simulink model "CP_DTSFC_Lin_b_n9945008"  (R2018b)
settings: Solver=FixedStepDiscrete  StartTime=0.0  StopTime=3  FixedStep=T_s  RelTol=1e-3
values from neighbouring files (symbols this model uses):
  Ad = sysdzoh.A    [CP_DTSFC_Lin_b_MainFile_n9945008.m]
  Bd = sysdzoh.B    [CP_DTSFC_Lin_b_MainFile_n9945008.m]
  Cd = sysdzoh.C    [CP_DTSFC_Lin_b_MainFile_n9945008.m]
  Dd = sysdzoh.D    [CP_DTSFC_Lin_b_MainFile_n9945008.m]
  K_db = place(sysdzoh.A ,sysdzoh.B ,dLambda)    [CP_DTSFC_Lin_b_MainFile_n9945008.m]
  T_s = 0.03    [CP_DTSFC_Lin_a_MainFile_n9945008.m]    (also in CP_DTSFC_Lin_b_MainFile_n9945008.m)
  x0 = [0.2 20*pi/180 0 0]'    [CP_DTSFC_Lin_a_MainFile_n9945008.m]    (also in CP_DTSFC_Lin_b_MainFile_n9945008.m)
settings Model: Creator=csmithcripps  LastModifiedBy=CodyS

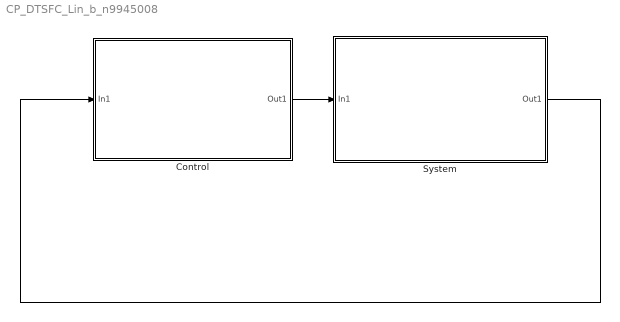
== system CP_DTSFC_Lin_b_n9945008 ==
  Control : Subsystem
  "System " : Subsystem
  wires:
  Control/1(Out1) -> "System "/1(In1)
  "System "/1(Out1) -> Control/1(In1)

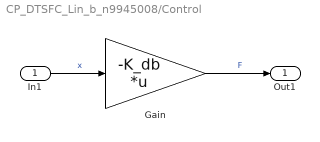
== system CP_DTSFC_Lin_b_n9945008/Control ==
  In1 : Inport
  Gain : Gain  Gain=-K_db  Multiplication=Matrix(K*u)
  Out1 : Outport
  wires:
  Gain/1 -> Out1/1  "F"
  In1/1 -> Gain/1  "x"

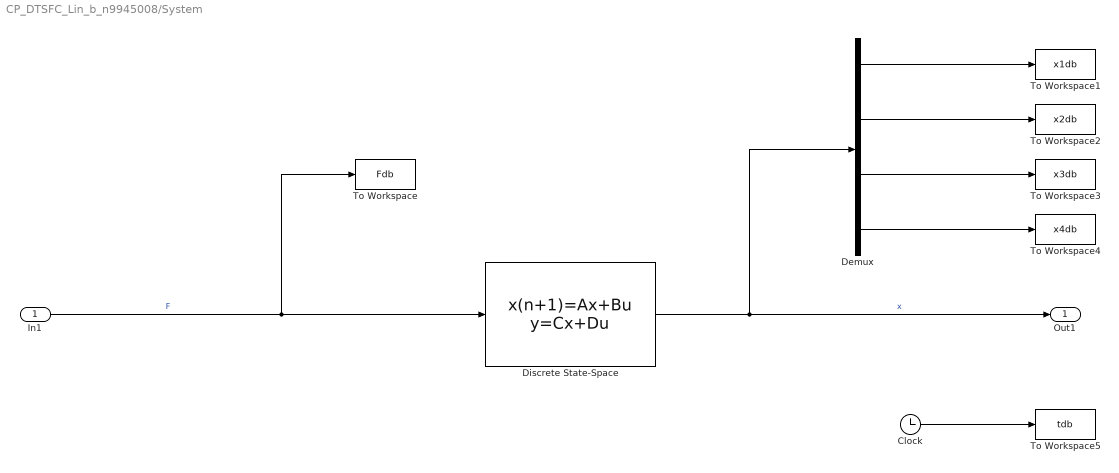
== system CP_DTSFC_Lin_b_n9945008/System  ==
  In1 : Inport
  Clock : Clock
  Demux : Demux
  Discrete State-Space : DiscreteStateSpace  A=Ad  B=Bd  C=Cd  D=Dd  InitialCondition=x0  SampleTime=T_s
  To Workspace : ToWorkspace  VariableName=Fdb  SampleTime=T_s
      settings: Save2DSignal=2-D array (concatenate along first dimension)
  To Workspace1 : ToWorkspace  VariableName=x1db  SampleTime=-1
      settings: Save2DSignal=2-D array (concatenate along first dimension)
  To Workspace2 : ToWorkspace  VariableName=x2db  SampleTime=-1
      settings: Save2DSignal=2-D array (concatenate along first dimension)
  To Workspace3 : ToWorkspace  VariableName=x3db  SampleTime=-1
      settings: Save2DSignal=2-D array (concatenate along first dimension)
  To Workspace4 : ToWorkspace  VariableName=x4db  SampleTime=-1
      settings: Save2DSignal=2-D array (concatenate along first dimension)
  To Workspace5 : ToWorkspace  VariableName=tdb  SampleTime=-1
      settings: Save2DSignal=2-D array (concatenate along first dimension)
  Out1 : Outport
  wires:
  In1/1 -> To Workspace/1, Discrete State-Space/1  "F"
  Demux/4 -> To Workspace4/1
  Demux/2 -> To Workspace2/1
  Demux/1 -> To Workspace1/1
  Demux/3 -> To Workspace3/1
  Clock/1 -> To Workspace5/1
  Discrete State-Space/1 -> Out1/1, Demux/1  "x"
